simulink model "sim_tcst_2024_att_ctrl"  (R2020a)
settings: Solver=ode4  StartTime=0.0  StopTime=30.0  FixedStep=0.01  RelTol=1e-3
values from neighbouring files (symbols this model uses):
  beta0 = 2    [init_tcst_2024_att_ctrl.m]
  c1_diff_sigma_bar_w = diag([12; 12; 12])    [init_tcst_2024_att_ctrl.m]
  c1_diff_ui = diag([25; 30; 20])    [init_tcst_2024_att_ctrl.m]
  c2_diff_sigma_bar_w = diag([12; 12; 12])    [init_tcst_2024_att_ctrl.m]
  c2_diff_ui = diag([50; 50; 10])    [init_tcst_2024_att_ctrl.m]
  c3_diff_sigma_bar_w = diag([15; 15; 15])    [init_tcst_2024_att_ctrl.m]
  c3_diff_ui = diag([15; 15; 10])    [init_tcst_2024_att_ctrl.m]
  dw_aa_t = 0.2 * ones(3, 5) + ( 1.0 - 0.2 ) * rand(3, 5)    [init_tcst_2024_att_ctrl.m]
  dw_ff_t = [ 0.4 * ones(1, 5) + ( 1.0 - 0.4 ) * rand(1, 5);                      0.4 * ones(1, 5) + ( 1.0 - 0.4 ) * rand(1, 5);                      0.2 * ones(1, 5) + ( 0.6 - 0.2 ) * rand(1, 5) ]    [init_tcst_2024_att_ctrl.m]
  dw_phi_t = ( - pi / 2 ) * ones(3, 5) + ( pi / 2 - ( - pi / 2 ) ) * rand(3, 5)    [init_tcst_2024_att_ctrl.m]
  dwci_init = zeros(3,5)    [init_tcst_2024_att_ctrl.m]
  err_Ri_bar_init = zeros(3,NF)    [init_tcst_2024_att_ctrl.m]
  Fi_init = zeros(3,NF)    [init_tcst_2024_att_ctrl.m]
  h1w = diag([20.0; 20.0; 20.0])    [init_tcst_2024_att_ctrl.m]
  h2w = diag([30.0; 35.0; 35.0])    [init_tcst_2024_att_ctrl.m]
  h3w = diag([30.0; 25.0; 30.0])    [init_tcst_2024_att_ctrl.m]
  Ji = zeros(3,3,NF)    [init_tcst_2024_att_ctrl.m]
  kr1 = 10    [init_tcst_2024_att_ctrl.m]
  kr2 = 10    [init_tcst_2024_att_ctrl.m]
  kr3 = 5    [init_tcst_2024_att_ctrl.m]
  Lamd_diff_sigma_bar_w = 0.8    [init_tcst_2024_att_ctrl.m]
  Lamd_diff_ui = 0.8    [init_tcst_2024_att_ctrl.m]
  mu_d_w = 100    [init_tcst_2024_att_ctrl.m]
  pos0 = zeros(3, 1)    [init_tcst_2024_att_ctrl.m]
  PZ0 = P0(3)    [init_tcst_2024_att_ctrl.m]
  PZ1 = 10    [init_tcst_2024_att_ctrl.m]
  Qci_init = repmat([1;0;0;0],1,NF)    [init_tcst_2024_att_ctrl.m]
  Qei_init = zeros(4,NF)    [init_tcst_2024_att_ctrl.m]
  R0 = 4    [init_tcst_2024_att_ctrl.m]
  R1 = 8    [init_tcst_2024_att_ctrl.m]
  Rci_init = zeros(3,3,NF)    [init_tcst_2024_att_ctrl.m]
  Rei_init = zeros(3,3,NF)    [init_tcst_2024_att_ctrl.m]
  Ri_init = zeros(3,3,NF)    [init_tcst_2024_att_ctrl.m]
  Rx2 = 10    [init_tcst_2024_att_ctrl.m]
  Ry2 = 6    [init_tcst_2024_att_ctrl.m]
  Rz2 = 4    [init_tcst_2024_att_ctrl.m]
  T0 = 0    [init_tcst_2024_att_ctrl.m]
  T1 = tseq1    (= 10)    [init_tcst_2024_att_ctrl.m]
  T2 = tseq1 + tseq12 + tseq2    (= 30)    [init_tcst_2024_att_ctrl.m]
  ui_init = zeros(3,NF)    [init_tcst_2024_att_ctrl.m]
  V_Phi_Rei_init = zeros(3,NF)    [init_tcst_2024_att_ctrl.m]
  vel0 = zeros(3, 1)    [init_tcst_2024_att_ctrl.m]
  wci_init = zeros(3,5)    [init_tcst_2024_att_ctrl.m]
  wei_init = zeros(3,NF)    [init_tcst_2024_att_ctrl.m]
  zeta_diff_sigma_bar_w = 0.3    [init_tcst_2024_att_ctrl.m]
  zeta_diff_ui = 0.05    [init_tcst_2024_att_ctrl.m]
undefined symbols (not defined in the file or in its folder): cal_frac_squ, p_alfaw1, p_alfaw2, q_alfaw1, q_alfaw2, Qi_init, wi_init
(part 4 of 4)

== matlab function sim_tcst_2024_att_ctrl/cal dw_hat agent 3 ==
  data: h3w input; Ji input; d_sigma_bar_w_vec input; sigma_bar_w_hat_vec input; dw_hat_3 output
function dw_hat_3 = fcn(h3w, Ji, d_sigma_bar_w_vec, sigma_bar_w_hat_vec)
%%%% 计算扰动观测值dw_hat
iiuav = 3;
dw_hat_3 = Ji(:,:,iiuav) * d_sigma_bar_w_vec(:,iiuav) + h3w * sigma_bar_w_hat_vec(:,iiuav);

== matlab function sim_tcst_2024_att_ctrl/cal dw_hat agent 4 ==
  data: h3w input; Ji input; d_sigma_bar_w_vec input; sigma_bar_w_hat_vec input; dw_hat_4 output
function dw_hat_4 = fcn(h3w, Ji, d_sigma_bar_w_vec, sigma_bar_w_hat_vec)
%%%% 计算扰动观测值dw_hat
iiuav = 4;
dw_hat_4 = Ji(:,:,iiuav) * d_sigma_bar_w_vec(:,iiuav) + h3w * sigma_bar_w_hat_vec(:,iiuav);

== matlab function sim_tcst_2024_att_ctrl/cal dw_hat agent 5 ==
  data: h3w input; Ji input; d_sigma_bar_w_vec input; sigma_bar_w_hat_vec input; dw_hat_5 output
function dw_hat_5 = fcn(h3w, Ji, d_sigma_bar_w_vec, sigma_bar_w_hat_vec)
%%%% 计算扰动观测值dw_hat
iiuav = 5;
dw_hat_5 = Ji(:,:,iiuav) * d_sigma_bar_w_vec(:,iiuav) + h3w * sigma_bar_w_hat_vec(:,iiuav);

== matlab function sim_tcst_2024_att_ctrl/cal Fi agent 1 ==
  data: wei_vec input; Rei_vec input; Fi_1 output; wci_vec input; dwci_vec input
function Fi_1 = fcn(wei_vec, Rei_vec, wci_vec, dwci_vec)
%%%% 计算辅助姿态旋转误差
iiuav = 1;
Fi_1 = cal_askew_mat( wei_vec(:,iiuav) ) * ( Rei_vec(:,:,iiuav)' ) * wci_vec(:,iiuav) ...
            - ( Rei_vec(:,:,iiuav)' ) * dwci_vec(:,iiuav);
end

== matlab function sim_tcst_2024_att_ctrl/cal error dw_tilt ==
  data: dw_vec input; dw_hat_vec input; dw_tilt_vec output
function dw_tilt_vec = fcn(dw_vec, dw_hat_vec)
%%%% 计算扰动观测误差dw_tilt
dw_tilt_vec = zeros(3,5);
for iiuav = 1:5
    dw_tilt_vec(:,iiuav) = dw_vec(:,iiuav) - dw_hat_vec(:,iiuav);
end

== matlab function sim_tcst_2024_att_ctrl/cal sigma_bar_w_hat agent 1 ==
  data: h1w input; h2w input; theta_sigma_bar_w_tilt_1_vec input; d_sigma_bar_w_hat_1 output; theta_sigma_bar_w_tilt_2_vec input; d_sigma_bar_w_vec input
function d_sigma_bar_w_hat_1 = fcn(h1w, h2w, theta_sigma_bar_w_tilt_1_vec, theta_sigma_bar_w_tilt_2_vec, d_sigma_bar_w_vec)
%%%% 计算扰动观测器中虚拟速度控制量观测值sigma_w_hat的微分方程
iiuav = 1;
d_sigma_bar_w_hat_1 = d_sigma_bar_w_vec(:,iiuav) + ...
                                            h1w * theta_sigma_bar_w_tilt_1_vec(:,iiuav) + ...
                                            h2w * theta_sigma_bar_w_tilt_2_vec(:,iiuav);

== matlab function sim_tcst_2024_att_ctrl/cal sigma_bar_w_hat agent 2 ==
  data: h1w input; h2w input; theta_sigma_bar_w_tilt_1_vec input; d_sigma_bar_w_hat_2 output; theta_sigma_bar_w_tilt_2_vec input; d_sigma_bar_w_vec input
function d_sigma_bar_w_hat_2 = fcn(h1w, h2w, theta_sigma_bar_w_tilt_1_vec, theta_sigma_bar_w_tilt_2_vec, d_sigma_bar_w_vec)
%%%% 计算扰动观测器中虚拟速度控制量观测值sigma_v_hat的微分方程
iiuav = 2;
d_sigma_bar_w_hat_2 = d_sigma_bar_w_vec(:,iiuav) + ...
                                            h1w * theta_sigma_bar_w_tilt_1_vec(:,iiuav) + ...
                                            h2w * theta_sigma_bar_w_tilt_2_vec(:,iiuav);

== matlab function sim_tcst_2024_att_ctrl/cal sigma_bar_w_hat agent 3 ==
  data: h1w input; h2w input; theta_sigma_bar_w_tilt_1_vec input; d_sigma_bar_w_hat_3 output; theta_sigma_bar_w_tilt_2_vec input; d_sigma_bar_w_vec input
function d_sigma_bar_w_hat_3 = fcn(h1w, h2w, theta_sigma_bar_w_tilt_1_vec, theta_sigma_bar_w_tilt_2_vec, d_sigma_bar_w_vec)
%%%% 计算扰动观测器中虚拟速度控制量观测值sigma_w_hat的微分方程
iiuav = 3;
d_sigma_bar_w_hat_3 = d_sigma_bar_w_vec(:,iiuav) + ...
                                            h1w * theta_sigma_bar_w_tilt_1_vec(:,iiuav) + ...
                                            h2w * theta_sigma_bar_w_tilt_2_vec(:,iiuav);

== matlab function sim_tcst_2024_att_ctrl/cal sigma_bar_w_hat agent 4 ==
  data: h1w input; h2w input; theta_sigma_bar_w_tilt_1_vec input; d_sigma_bar_w_hat_4 output; theta_sigma_bar_w_tilt_2_vec input; d_sigma_bar_w_vec input
function d_sigma_bar_w_hat_4 = fcn(h1w, h2w, theta_sigma_bar_w_tilt_1_vec, theta_sigma_bar_w_tilt_2_vec, d_sigma_bar_w_vec)
%%%% 计算扰动观测器中虚拟速度控制量观测值sigma_w_hat的微分方程
iiuav = 4;
d_sigma_bar_w_hat_4 = d_sigma_bar_w_vec(:,iiuav) + ...
                                            h1w * theta_sigma_bar_w_tilt_1_vec(:,iiuav) + ...
                                            h2w * theta_sigma_bar_w_tilt_2_vec(:,iiuav);

== matlab function sim_tcst_2024_att_ctrl/cal sigma_bar_w_hat agent 5 ==
  data: h1w input; h2w input; theta_sigma_bar_w_tilt_1_vec input; d_sigma_bar_w_hat_5 output; theta_sigma_bar_w_tilt_2_vec input; d_sigma_bar_w_vec input
function d_sigma_bar_w_hat_5 = fcn(h1w, h2w, theta_sigma_bar_w_tilt_1_vec, theta_sigma_bar_w_tilt_2_vec, d_sigma_bar_w_vec)
%%%% 计算扰动观测器中虚拟速度控制量观测值sigma_w_hat的微分方程
iiuav = 5;
d_sigma_bar_w_hat_5 = d_sigma_bar_w_vec(:,iiuav) + ...
                                            h1w * theta_sigma_bar_w_tilt_1_vec(:,iiuav) + ...
                                            h2w * theta_sigma_bar_w_tilt_2_vec(:,iiuav);

== matlab function sim_tcst_2024_att_ctrl/cal sigma_w_bar ==
  data: sigma_bar_w_vec output; wi_vec input; sigma_w_vec input
function sigma_bar_w_vec = fcn(wi_vec, sigma_w_vec)
%%%% 计算姿态角速率跟踪误差
sigma_bar_w_vec = zeros(3,5);
for iiuav = 1:5
    sigma_bar_w_vec(:,iiuav) = wi_vec(:,iiuav) - sigma_w_vec(:,iiuav);
end

== matlab function sim_tcst_2024_att_ctrl/cal theta_sigma_bar_w_tilt agent 1 ==
  data: alfa_theta_obs_w input; sigma_bar_w_tilt_squ_1_1 input; theta_sigma_bar_w_tilt_1_1 output; sigma_bar_w_tilt_squ_2_1 input; sigma_bar_w_tilt_vec input; theta_sigma_bar_w_tilt_2_1 output
function [theta_sigma_bar_w_tilt_1_1, theta_sigma_bar_w_tilt_2_1] = fcn(alfa_theta_obs_w, sigma_bar_w_tilt_squ_1_1, sigma_bar_w_tilt_squ_2_1, sigma_bar_w_tilt_vec)
%%%% 计算平滑递增函数
iiuav = 1;
theta_sigma_bar_w_tilt_1_1 = sigma_bar_w_tilt_squ_1_1(:) .* ( -1 + 2 ./ ( 1 + exp( -alfa_theta_obs_w .* sigma_bar_w_tilt_vec(:,iiuav) ) ) );
theta_sigma_bar_w_tilt_2_1 = sigma_bar_w_tilt_squ_2_1(:) .* ( -1 + 2 ./ ( 1 + exp( -alfa_theta_obs_w .* sigma_bar_w_tilt_vec(:,iiuav) ) ) );

== matlab function sim_tcst_2024_att_ctrl/cal theta_sigma_bar_w_tilt agent 2 ==
  data: alfa_theta_obs_w input; sigma_bar_w_tilt_squ_1_2 input; theta_sigma_bar_w_tilt_1_2 output; sigma_bar_w_tilt_squ_2_2 input; sigma_bar_w_tilt_vec input; theta_sigma_bar_w_tilt_2_2 output
function [theta_sigma_bar_w_tilt_1_2, theta_sigma_bar_w_tilt_2_2] = fcn(alfa_theta_obs_w, sigma_bar_w_tilt_squ_1_2, sigma_bar_w_tilt_squ_2_2, sigma_bar_w_tilt_vec)
%%%% 计算平滑递增函数
iiuav = 2;
theta_sigma_bar_w_tilt_1_2 = sigma_bar_w_tilt_squ_1_2(:) .* ( -1 + 2 ./ ( 1 + exp( -alfa_theta_obs_w .* sigma_bar_w_tilt_vec(:,iiuav) ) ) );
theta_sigma_bar_w_tilt_2_2 = sigma_bar_w_tilt_squ_2_2(:) .* ( -1 + 2 ./ ( 1 + exp( -alfa_theta_obs_w .* sigma_bar_w_tilt_vec(:,iiuav) ) ) );

== matlab function sim_tcst_2024_att_ctrl/cal Fi agent 2 ==
  data: wei_vec input; Rei_vec input; Fi_2 output; wci_vec input; dwci_vec input
function Fi_2 = fcn(wei_vec, Rei_vec, wci_vec, dwci_vec)
%%%% 计算辅助姿态旋转误差
iiuav = 2;
Fi_2 = cal_askew_mat( wei_vec(:,iiuav) ) * ( Rei_vec(:,:,iiuav)' ) * wci_vec(:,iiuav) ...
            - ( Rei_vec(:,:,iiuav)' ) * dwci_vec(:,iiuav);
end

== matlab function sim_tcst_2024_att_ctrl/cal theta_sigma_bar_w_tilt agent 3 ==
  data: alfa_theta_obs_w input; sigma_bar_w_tilt_squ_1_3 input; theta_sigma_bar_w_tilt_1_3 output; sigma_bar_w_tilt_squ_2_3 input; sigma_bar_w_tilt_vec input; theta_sigma_bar_w_tilt_2_3 output
function [theta_sigma_bar_w_tilt_1_3, theta_sigma_bar_w_tilt_2_3] = fcn(alfa_theta_obs_w, sigma_bar_w_tilt_squ_1_3, sigma_bar_w_tilt_squ_2_3, sigma_bar_w_tilt_vec)
%%%% 计算平滑递增函数
iiuav = 3;
theta_sigma_bar_w_tilt_1_3 = sigma_bar_w_tilt_squ_1_3(:) .* ( -1 + 2 ./ ( 1 + exp( -alfa_theta_obs_w .* sigma_bar_w_tilt_vec(:,iiuav) ) ) );
theta_sigma_bar_w_tilt_2_3 = sigma_bar_w_tilt_squ_2_3(:) .* ( -1 + 2 ./ ( 1 + exp( -alfa_theta_obs_w .* sigma_bar_w_tilt_vec(:,iiuav) ) ) );

== matlab function sim_tcst_2024_att_ctrl/cal theta_sigma_bar_w_tilt agent 4 ==
  data: alfa_theta_obs_w input; sigma_bar_w_tilt_squ_1_4 input; theta_sigma_bar_w_tilt_1_4 output; sigma_bar_w_tilt_squ_2_4 input; sigma_bar_w_tilt_vec input; theta_sigma_bar_w_tilt_2_4 output
function [theta_sigma_bar_w_tilt_1_4, theta_sigma_bar_w_tilt_2_4] = fcn(alfa_theta_obs_w, sigma_bar_w_tilt_squ_1_4, sigma_bar_w_tilt_squ_2_4, sigma_bar_w_tilt_vec)
%%%% 计算平滑递增函数
iiuav = 4;
theta_sigma_bar_w_tilt_1_4 = sigma_bar_w_tilt_squ_1_4(:) .* ( -1 + 2 ./ ( 1 + exp( -alfa_theta_obs_w .* sigma_bar_w_tilt_vec(:,iiuav) ) ) );
theta_sigma_bar_w_tilt_2_4 = sigma_bar_w_tilt_squ_2_4(:) .* ( -1 + 2 ./ ( 1 + exp( -alfa_theta_obs_w .* sigma_bar_w_tilt_vec(:,iiuav) ) ) );

== matlab function sim_tcst_2024_att_ctrl/cal theta_sigma_bar_w_tilt agent 5 ==
  data: alfa_theta_obs_w input; sigma_bar_w_tilt_squ_1_5 input; theta_sigma_bar_w_tilt_1_5 output; sigma_bar_w_tilt_squ_2_5 input; sigma_bar_w_tilt_vec input; theta_sigma_bar_w_tilt_2_5 output
function [theta_sigma_bar_w_tilt_1_5, theta_sigma_bar_w_tilt_2_5] = fcn(alfa_theta_obs_w, sigma_bar_w_tilt_squ_1_5, sigma_bar_w_tilt_squ_2_5, sigma_bar_w_tilt_vec)
%%%% 计算平滑递增函数
iiuav = 5;
theta_sigma_bar_w_tilt_1_5 = sigma_bar_w_tilt_squ_1_5(:) .* ( -1 + 2 ./ ( 1 + exp( -alfa_theta_obs_w .* sigma_bar_w_tilt_vec(:,iiuav) ) ) );
theta_sigma_bar_w_tilt_2_5 = sigma_bar_w_tilt_squ_2_5(:) .* ( -1 + 2 ./ ( 1 + exp( -alfa_theta_obs_w .* sigma_bar_w_tilt_vec(:,iiuav) ) ) );

== matlab function sim_tcst_2024_att_ctrl/choose ksi_est_err 11 ==
  data: x input; y output
function y = fcn(x)
iiuav = 1;
y = x(:,iiuav);

== matlab function sim_tcst_2024_att_ctrl/choose ksi_est_err 12 ==
  data: x input; y output
function y = fcn(x)
iiuav = 1;
y = x(:,iiuav);

== matlab function sim_tcst_2024_att_ctrl/choose ksi_est_err 13 ==
  data: x input; y output
function y = fcn(x)
iiuav = 2;
y = x(:,iiuav);

== matlab function sim_tcst_2024_att_ctrl/choose ksi_est_err 14 ==
  data: x input; y output
function y = fcn(x)
iiuav = 2;
y = x(:,iiuav);

== matlab function sim_tcst_2024_att_ctrl/choose ksi_est_err 15 ==
  data: x input; y output
function y = fcn(x)
iiuav = 3;
y = x(:,iiuav);

== matlab function sim_tcst_2024_att_ctrl/choose ksi_est_err 16 ==
  data: x input; y output
function y = fcn(x)
iiuav = 3;
y = x(:,iiuav);

== matlab function sim_tcst_2024_att_ctrl/choose ksi_est_err 17 ==
  data: x input; y output
function y = fcn(x)
iiuav = 4;
y = x(:,iiuav);

== matlab function sim_tcst_2024_att_ctrl/choose ksi_est_err 18 ==
  data: x input; y output
function y = fcn(x)
iiuav = 4;
y = x(:,iiuav);

== matlab function sim_tcst_2024_att_ctrl/choose ksi_est_err 19 ==
  data: x input; y output
function y = fcn(x)
iiuav = 5;
y = x(:,iiuav);

== matlab function sim_tcst_2024_att_ctrl/choose ksi_est_err 20 ==
  data: x input; y output
function y = fcn(x)
iiuav = 5;
y = x(:,iiuav);

== matlab function sim_tcst_2024_att_ctrl/cal Fi agent 3 ==
  data: wei_vec input; Rei_vec input; Fi_3 output; wci_vec input; dwci_vec input
function Fi_3 = fcn(wei_vec, Rei_vec, wci_vec, dwci_vec)
%%%% 计算辅助姿态旋转误差
iiuav = 3;
Fi_3 = cal_askew_mat( wei_vec(:,iiuav) ) * ( Rei_vec(:,:,iiuav)' ) * wci_vec(:,iiuav) ...
            - ( Rei_vec(:,:,iiuav)' ) * dwci_vec(:,iiuav);
end

== matlab function sim_tcst_2024_att_ctrl/combine d_sigma_bar_v_est ==
  data: d_sigma_bar_w_est_1 input; d_sigma_bar_w_est_2 input; d_sigma_bar_w_est_3 input; d_sigma_bar_w_est_4 input; d_sigma_bar_w_est_5 input; d_sigma_bar_w_vec output
function d_sigma_bar_w_vec  = fcn(d_sigma_bar_w_est_1, d_sigma_bar_w_est_2, d_sigma_bar_w_est_3, d_sigma_bar_w_est_4, d_sigma_bar_w_est_5)
%%%% 合并用微分器求得的虚拟速度控制量导数
d_sigma_bar_w_vec = [d_sigma_bar_w_est_1(:), d_sigma_bar_w_est_2(:), d_sigma_bar_w_est_3(:), d_sigma_bar_w_est_4(:), d_sigma_bar_w_est_5(:)];

== matlab function sim_tcst_2024_att_ctrl/combine dw_hat ==
  data: dw_hat_1 input; dw_hat_2 input; dw_hat_3 input; dw_hat_4 input; dw_hat_5 input; dw_hat_vec output
function dw_hat_vec  = fcn(dw_hat_1, dw_hat_2, dw_hat_3, dw_hat_4, dw_hat_5)
%%%% 合并扰动观测值dw_hat
dw_hat_vec = [dw_hat_1(:), dw_hat_2(:), dw_hat_3(:), dw_hat_4(:), dw_hat_5(:)];

== matlab function sim_tcst_2024_att_ctrl/combine sigma_bar_w_hat ==
  data: sigma_bar_w_hat_1 input; sigma_bar_w_hat_2 input; sigma_bar_w_hat_3 input; sigma_bar_w_hat_4 input; sigma_bar_w_hat_5 input; sigma_bar_w_hat_vec output
function sigma_bar_w_hat_vec  = fcn(sigma_bar_w_hat_1, sigma_bar_w_hat_2, sigma_bar_w_hat_3, sigma_bar_w_hat_4, sigma_bar_w_hat_5)
%%%% 合并虚拟速度控制量观测值sigma_bar_w_hat
sigma_bar_w_hat_vec = [sigma_bar_w_hat_1(:), sigma_bar_w_hat_2(:), sigma_bar_w_hat_3(:), sigma_bar_w_hat_4(:), sigma_bar_w_hat_5(:)];

== matlab function sim_tcst_2024_att_ctrl/combine sigma_w ==
  data: sigma_w_1 input; sigma_w_vec output; sigma_w_2 input; sigma_w_3 input; sigma_w_4 input; sigma_w_5 input
function sigma_w_vec = fcn(sigma_w_1, sigma_w_2, sigma_w_3, sigma_w_4, sigma_w_5)
%%%% 合并辅助姿态角速率
sigma_w_vec = [sigma_w_1(:), sigma_w_2(:), sigma_w_3(:), sigma_w_4(:), sigma_w_5(:)];

== matlab function sim_tcst_2024_att_ctrl/combine theta_sigma_bar_w_tilt ==
  data: theta_sigma_bar_w_tilt_1_1 input; theta_sigma_bar_w_tilt_1_2 input; theta_sigma_bar_w_tilt_1_3 input; theta_sigma_bar_w_tilt_1_4 input; theta_sigma_bar_w_tilt_1_5 input; theta_sigma_bar_w_tilt_1_vec output; theta_sigma_bar_w_tilt_2_1 input; theta_sigma_bar_w_tilt_2_vec output; theta_sigma_bar_w_tilt_2_2 input; theta_sigma_bar_w_tilt_2_3 input; theta_sigma_bar_w_tilt_2_4 input; theta_sigma_bar_w_tilt_2_5 input
function [theta_sigma_bar_w_tilt_1_vec, theta_sigma_bar_w_tilt_2_vec]  = fcn(theta_sigma_bar_w_tilt_1_1, theta_sigma_bar_w_tilt_1_2, theta_sigma_bar_w_tilt_1_3, theta_sigma_bar_w_tilt_1_4, theta_sigma_bar_w_tilt_1_5, ...
                                                                                                                                            theta_sigma_bar_w_tilt_2_1, theta_sigma_bar_w_tilt_2_2, theta_sigma_bar_w_tilt_2_3, theta_sigma_bar_w_tilt_2_4, theta_sigma_bar_w_tilt_2_5)
%%%% 合并领导者位置观测器输出结果
theta_sigma_bar_w_tilt_1_vec = [theta_sigma_bar_w_tilt_1_1(:), theta_sigma_bar_w_tilt_1_2(:), theta_sigma_bar_w_tilt_1_3(:), theta_sigma_bar_w_tilt_1_4(:), theta_sigma_bar_w_tilt_1_5(:)];
theta_sigma_bar_w_tilt_2_vec = [theta_sigma_bar_w_tilt_2_1(:), theta_sigma_bar_w_tilt_2_2(:), theta_sigma_bar_w_tilt_2_3(:), theta_sigma_bar_w_tilt_2_4(:), theta_sigma_bar_w_tilt_2_5(:)];

== matlab function sim_tcst_2024_att_ctrl/trans to column51 ==
  data: x input; y output
function y = fcn(x)
y = x(:);

== matlab function sim_tcst_2024_att_ctrl/trans to column52 ==
  data: x input; y output
function y = fcn(x)
y = x(:);

== matlab function sim_tcst_2024_att_ctrl/trans to column53 ==
  data: x input; y output
function y = fcn(x)
y = x(:);

== matlab function sim_tcst_2024_att_ctrl/trans to column54 ==
  data: x input; y output
function y = fcn(x)
y = x(:);

== matlab function sim_tcst_2024_att_ctrl/trans to column55 ==
  data: x input; y output
function y = fcn(x)
y = x(:);

== matlab function sim_tcst_2024_att_ctrl/trans to column56 ==
  data: x input; y output
function y = fcn(x)
y = x(:);

== matlab function sim_tcst_2024_att_ctrl/cal Fi agent 4 ==
  data: wei_vec input; Rei_vec input; Fi_4 output; wci_vec input; dwci_vec input
function Fi_4 = fcn(wei_vec, Rei_vec, wci_vec, dwci_vec)
%%%% 计算辅助姿态旋转误差
iiuav = 4;
Fi_4 = cal_askew_mat( wei_vec(:,iiuav) ) * ( Rei_vec(:,:,iiuav)' ) * wci_vec(:,iiuav) ...
            - ( Rei_vec(:,:,iiuav)' ) * dwci_vec(:,iiuav);
end

== matlab function sim_tcst_2024_att_ctrl/trans to column57 ==
  data: x input; y output
function y = fcn(x)
y = x(:);

== matlab function sim_tcst_2024_att_ctrl/trans to column58 ==
  data: x input; y output
function y = fcn(x)
y = x(:);

== matlab function sim_tcst_2024_att_ctrl/trans to column59 ==
  data: x input; y output
function y = fcn(x)
y = x(:);

== matlab function sim_tcst_2024_att_ctrl/trans to column60 ==
  data: x input; y output
function y = fcn(x)
y = x(:);

== matlab function sim_tcst_2024_att_ctrl/combine tau1 ==
  data: dw_1 input; dw_vec output; dw_2 input; dw_3 input; dw_4 input; dw_5 input
function dw_vec = fcn(dw_1, dw_2, dw_3, dw_4, dw_5)
%%%% 合并辅助姿态角速率
dw_vec = [dw_1(:), dw_2(:), dw_3(:), dw_4(:), dw_5(:)];

== matlab function sim_tcst_2024_att_ctrl/generate angular rate disturbance agent 1 ==
  data: dw_1 output; dw_aa_t input; dw_ff_t input; dw_phi_t input; t input
function dw_1 = fcn(dw_aa_t, dw_ff_t, dw_phi_t, t)
%%%% 姿态动力学方程中的扰动项设置
epsil_t = zeros(3, 1);

for kk = 1:5
    epsil_t = epsil_t + dw_aa_t(:, kk) .* sin( 2 * pi * dw_ff_t(:, kk) * t + dw_phi_t(:, kk) );
end

dw_1 = [ epsil_t(1) + 1.6 * sin( 0.4 * t ) + 2.0 * cos( 0.5 * t ) + 1.4 * sin( 0.7 * t ) ...
                + 4 * exp( -0.1 * t ) * sin( 0.8 * t ) + 3 / ( 1 + exp( -0.2 * ( t - 15 ) ) ); ...
                epsil_t(2) + 1.2 * sin( 0.2 * t ) + 3 * cos( 0.4 * t ) + 0.8 * sin( 0.6 * t ) ...
                + 2 * exp( -0.15 * t ) * cos( 1.2 * t ) + 3 / ( 1 + exp( -0.3 * ( t - 25 ) ) ); ...
                epsil_t(3) + 1.8 * sin( 0.2 * t ) + 1.6 * sin( 0.3 * t ) + 1.6 * cos( 0.4 * t ) ...
                + 4 * exp( -0.05 * t ) * sin( 0.5 * t + pi / 4 ) + 3 / ( 1 + exp( -0.5 * ( t - 20 ) ) ) ];

== matlab function sim_tcst_2024_att_ctrl/generate angular rate disturbance agent 2 ==
  data: dw_2 output; dw_aa_t input; dw_ff_t input; dw_phi_t input; t input
function dw_2 = fcn(dw_aa_t, dw_ff_t, dw_phi_t, t)
%%%% 姿态动力学方程中的扰动项设置
epsil_t = zeros(3, 1);

for kk = 1:5
    epsil_t = epsil_t + dw_aa_t(:, kk) .* sin( 2 * pi * dw_ff_t(:, kk) * t + dw_phi_t(:, kk) );
end

dw_2 = [ epsil_t(1) + 1.6 * sin( 0.2 * t ) + 2.0 * cos( 0.3 * t ) + 1.4 * sin( 0.5 * t ) ...
                + 4 * exp( -0.1 * t ) * sin( 0.5 * t ) + 3 / ( 1 + exp( -0.2 * ( t - 15 ) ) ); ...
                epsil_t(2) + 1.2 * sin( 0.1 * t ) + 3 * cos( 0.2 * t ) + 0.8 * sin( 0.4 * t ) ...
                + 2 * exp( -0.15 * t ) * cos( 0.6 * t ) + 3 / ( 1 + exp( -0.3 * ( t - 25 ) ) ); ...
                epsil_t(3) + 1.8 * sin( 0.1 * t ) + 1.6 * sin( 0.2 * t ) + 1.6 * cos( 0.3 * t ) ...
                + 4 * exp( -0.05 * t ) * sin( 0.4 * t + pi / 4 ) + 3 / ( 1 + exp( -0.5 * ( t - 20 ) ) ) ];

== matlab function sim_tcst_2024_att_ctrl/generate angular rate disturbance agent 3 ==
  data: dw_3 output; dw_aa_t input; dw_ff_t input; dw_phi_t input; t input
function dw_3 = fcn(dw_aa_t, dw_ff_t, dw_phi_t, t)
%%%% 姿态动力学方程中的扰动项设置
epsil_t = zeros(3, 1);

for kk = 1:5
    epsil_t = epsil_t + dw_aa_t(:, kk) .* sin( 2 * pi * dw_ff_t(:, kk) * t + dw_phi_t(:, kk) );
end

dw_3 = [ epsil_t(1) + 1.6 * sin( 0.2 * t ) + 2.0 * cos( 0.3 * t ) + 1.4 * sin( 0.5 * t ) ...
                + 4 * exp( -0.1 * t ) * sin( 0.5 * t ) + 3 / ( 1 + exp( -0.2 * ( t - 15 ) ) ); ...
                epsil_t(2) + 1.2 * sin( 0.1 * t ) + 3 * cos( 0.2 * t ) + 0.8 * sin( 0.4 * t ) ...
                + 2 * exp( -0.15 * t ) * cos( 0.6 * t ) + 3 / ( 1 + exp( -0.3 * ( t - 25 ) ) ); ...
                epsil_t(3) + 1.8 * sin( 0.1 * t ) + 1.6 * sin( 0.2 * t ) + 1.6 * cos( 0.3 * t ) ...
                + 4 * exp( -0.05 * t ) * sin( 0.4 * t + pi / 4 ) + 3 / ( 1 + exp( -0.5 * ( t - 20 ) ) ) ];

== matlab function sim_tcst_2024_att_ctrl/generate angular rate disturbance agent 4 ==
  data: dw_4 output; dw_aa_t input; dw_ff_t input; dw_phi_t input; t input
function dw_4 = fcn(dw_aa_t, dw_ff_t, dw_phi_t, t)
%%%% 姿态动力学方程中的扰动项设置
epsil_t = zeros(3, 1);

for kk = 1:5
    epsil_t = epsil_t + dw_aa_t(:, kk) .* sin( 2 * pi * dw_ff_t(:, kk) * t + dw_phi_t(:, kk) );
end

dw_4 = [ epsil_t(1) + 1.6 * sin( 0.2 * t ) + 2.0 * cos( 0.3 * t ) + 1.4 * sin( 0.5 * t ) ...
                + 4 * exp( -0.1 * t ) * sin( 0.5 * t ) + 3 / ( 1 + exp( -0.2 * ( t - 15 ) ) ); ...
                epsil_t(2) + 1.2 * sin( 0.1 * t ) + 3 * cos( 0.2 * t ) + 0.8 * sin( 0.4 * t ) ...
                + 2 * exp( -0.15 * t ) * cos( 0.6 * t ) + 3 / ( 1 + exp( -0.3 * ( t - 25 ) ) ); ...
                epsil_t(3) + 1.8 * sin( 0.1 * t ) + 1.6 * sin( 0.2 * t ) + 1.6 * cos( 0.3 * t ) ...
                + 4 * exp( -0.05 * t ) * sin( 0.4 * t + pi / 4 ) + 3 / ( 1 + exp( -0.5 * ( t - 20 ) ) ) ];

== matlab function sim_tcst_2024_att_ctrl/generate angular rate disturbance agent 5 ==
  data: dw_5 output; dw_aa_t input; dw_ff_t input; dw_phi_t input; t input
function dw_5 = fcn(dw_aa_t, dw_ff_t, dw_phi_t, t)
%%%% 姿态动力学方程中的扰动项设置
epsil_t = zeros(3, 1);

for kk = 1:5
    epsil_t = epsil_t + dw_aa_t(:, kk) .* sin( 2 * pi * dw_ff_t(:, kk) * t + dw_phi_t(:, kk) );
end

dw_5 = [ epsil_t(1) + 1.6 * sin( 0.2 * t ) + 2.0 * cos( 0.3 * t ) + 1.4 * sin( 0.5 * t ) ...
                + 4 * exp( -0.1 * t ) * sin( 0.5 * t ) + 3 / ( 1 + exp( -0.2 * ( t - 15 ) ) ); ...
                epsil_t(2) + 1.2 * sin( 0.1 * t ) + 3 * cos( 0.2 * t ) + 0.8 * sin( 0.4 * t ) ...
                + 2 * exp( -0.15 * t ) * cos( 0.6 * t ) + 3 / ( 1 + exp( -0.3 * ( t - 25 ) ) ); ...
                epsil_t(3) + 1.8 * sin( 0.1 * t ) + 1.6 * sin( 0.2 * t ) + 1.6 * cos( 0.3 * t ) ...
                + 4 * exp( -0.05 * t ) * sin( 0.4 * t + pi / 4 ) + 3 / ( 1 + exp( -0.5 * ( t - 20 ) ) ) ];

== matlab function sim_tcst_2024_att_ctrl/combine norminal formation control input ==
  data: ui_1 input; ui_vec output; ui_2 input; ui_3 input; ui_4 input; ui_5 input
function ui_vec = fcn(ui_1, ui_2, ui_3, ui_4, ui_5)
%%%% 合并领导者编队跟踪误差结果
ui_vec = [ui_1(:), ui_2(:), ui_3(:), ui_4(:), ui_5(:)];

== matlab function sim_tcst_2024_att_ctrl/cal Fi agent 5 ==
  data: wei_vec input; Rei_vec input; Fi_5 output; wci_vec input; dwci_vec input
function Fi_5 = fcn(wei_vec, Rei_vec, wci_vec, dwci_vec)
%%%% 计算辅助姿态旋转误差
iiuav = 5;
Fi_5 = cal_askew_mat( wei_vec(:,iiuav) ) * ( Rei_vec(:,:,iiuav)' ) * wci_vec(:,iiuav) ...
            - ( Rei_vec(:,:,iiuav)' ) * dwci_vec(:,iiuav);
end

== matlab function sim_tcst_2024_att_ctrl/control input generator agent 1 ==
  data: u0 input; ui output
function ui  = fcn(u0)
%%%% 给出领导者参考加速度控制输入
g0 = 9.80663;
e3 = [0;0;1];

ui = g0 * e3 + u0(:);

== matlab function sim_tcst_2024_att_ctrl/control input generator agent 2 ==
  data: u0 input; ui output
function ui  = fcn(u0)
%%%% 给出领导者参考加速度控制输入
g0 = 9.80663;
e3 = [0;0;1];

ui = g0 * e3 + u0(:);

== matlab function sim_tcst_2024_att_ctrl/control input generator agent 3 ==
  data: u0 input; ui output
function ui  = fcn(u0)
%%%% 给出领导者参考加速度控制输入
g0 = 9.80663;
e3 = [0;0;1];

ui = g0 * e3 + u0(:);

== matlab function sim_tcst_2024_att_ctrl/control input generator agent 4 ==
  data: u0 input; ui output
function ui  = fcn(u0)
%%%% 给出领导者参考加速度控制输入
g0 = 9.80663;
e3 = [0;0;1];

ui = g0 * e3 + u0(:);

== matlab function sim_tcst_2024_att_ctrl/control input generator agent 5 ==
  data: u0 input; ui output
function ui  = fcn(u0)
%%%% 给出领导者参考加速度控制输入
g0 = 9.80663;
e3 = [0;0;1];

ui = g0 * e3 + u0(:);

== matlab function sim_tcst_2024_att_ctrl/combine err_Ri_bar1 ==
  data: Fi_1 input; Fi_vec output; Fi_2 input; Fi_3 input; Fi_4 input; Fi_5 input
function Fi_vec = fcn(Fi_1, Fi_2, Fi_3, Fi_4, Fi_5)
%%%% 合并补偿函数向量
Fi_vec = [Fi_1(:), Fi_2(:), Fi_3(:), Fi_4(:), Fi_5(:)];

== matlab function sim_tcst_2024_att_ctrl/update VTi agent 1 ==
  data: kr2 input; kr3 input; d_VTi_1 output; beta0 input; err_Ri_bar_vec input
function d_VTi_1 = fcn(kr2, kr3, beta0, err_Ri_bar_vec)
%%%% 更新非线性Filippov解向量
iiuav = 1;
d_VTi_1 = kr3 * kr2 * err_Ri_bar_vec(:,iiuav) - beta0 * sign( err_Ri_bar_vec(:,iiuav) );
end

== matlab function sim_tcst_2024_att_ctrl/update VTi agent 2 ==
  data: kr2 input; kr3 input; d_VTi_2 output; beta0 input; err_Ri_bar_vec input
function d_VTi_2 = fcn(kr2, kr3, beta0, err_Ri_bar_vec)
%%%% 更新非线性Filippov解向量
iiuav = 2;
d_VTi_2 = kr3 * kr2 * err_Ri_bar_vec(:,iiuav) - beta0 * sign( err_Ri_bar_vec(:,iiuav) );
end

== matlab function sim_tcst_2024_att_ctrl/update VTi agent 3 ==
  data: kr2 input; kr3 input; d_VTi_3 output; beta0 input; err_Ri_bar_vec input
function d_VTi_3 = fcn(kr2, kr3, beta0, err_Ri_bar_vec)
%%%% 更新非线性Filippov解向量
iiuav = 3;
d_VTi_3 = kr3 * kr2 * err_Ri_bar_vec(:,iiuav) - beta0 * sign( err_Ri_bar_vec(:,iiuav) );
end

== matlab function sim_tcst_2024_att_ctrl/update VTi agent 4 ==
  data: kr2 input; kr3 input; d_VTi_4 output; beta0 input; err_Ri_bar_vec input
function d_VTi_4 = fcn(kr2, kr3, beta0, err_Ri_bar_vec)
%%%% 更新非线性Filippov解向量
iiuav = 4;
d_VTi_4 = kr3 * kr2 * err_Ri_bar_vec(:,iiuav) - beta0 * sign( err_Ri_bar_vec(:,iiuav) );
end

== matlab function sim_tcst_2024_att_ctrl/update VTi agent 5 ==
  data: kr2 input; kr3 input; d_VTi_5 output; beta0 input; err_Ri_bar_vec input
function d_VTi_5 = fcn(kr2, kr3, beta0, err_Ri_bar_vec)
%%%% 更新非线性Filippov解向量
iiuav = 5;
d_VTi_5 = kr3 * kr2 * err_Ri_bar_vec(:,iiuav) - beta0 * sign( err_Ri_bar_vec(:,iiuav) );
end

== matlab function sim_tcst_2024_att_ctrl/combine VTi ==
  data: VTi_1 input; VTi_vec output; VTi_2 input; VTi_3 input; VTi_4 input; VTi_5 input
function VTi_vec = fcn(VTi_1, VTi_2, VTi_3, VTi_4, VTi_5)
%%%% 合并非线性Filippov解向量
VTi_vec = [VTi_1(:), VTi_2(:), VTi_3(:), VTi_4(:), VTi_5(:)];

== matlab function sim_tcst_2024_att_ctrl/cal taui agent 2 ==
  data: kr1 input; kr2 input; kr3 input; tau_2 output; Ji input; wi_vec input; wei_vec input; err_Ri_bar_vec input; Fi_vec input; VTi_vec input; dw_hat_vec input
function tau_2 = fcn(kr1, kr2, kr3, Ji, wi_vec, wei_vec, err_Ri_bar_vec, Fi_vec, VTi_vec, dw_hat_vec)
%%%% 计算用于姿态控制的驱动力矩控制输入
iiuav = 2;
tau_2 = -( kr3 + kr2 ) * err_Ri_bar_vec(:,iiuav) - kr1 * Ji(:,:,iiuav) * wei_vec(:,iiuav) ...
                + cal_askew_mat( wi_vec(:,iiuav) ) * Ji(:,:,iiuav) * wi_vec(:,iiuav) ...
                - Ji(:,:,iiuav) * Fi_vec(:,iiuav) - dw_hat_vec(:,iiuav) - VTi_vec(:,iiuav);
end

== matlab function sim_tcst_2024_att_ctrl/cal taui agent 3 ==
  data: kr1 input; kr2 input; kr3 input; tau_3 output; Ji input; wi_vec input; wei_vec input; err_Ri_bar_vec input; Fi_vec input; VTi_vec input; dw_hat_vec input
function tau_3 = fcn(kr1, kr2, kr3, Ji, wi_vec, wei_vec, err_Ri_bar_vec, Fi_vec, VTi_vec, dw_hat_vec)
%%%% 计算用于姿态控制的驱动力矩控制输入
iiuav = 3;
tau_3 = -( kr3 + kr2 ) * err_Ri_bar_vec(:,iiuav) - kr1 * Ji(:,:,iiuav) * wei_vec(:,iiuav) ...
                + cal_askew_mat( wi_vec(:,iiuav) ) * Ji(:,:,iiuav) * wi_vec(:,iiuav) ...
                - Ji(:,:,iiuav) * Fi_vec(:,iiuav) - dw_hat_vec(:,iiuav) - VTi_vec(:,iiuav);
end

== matlab function sim_tcst_2024_att_ctrl/cal taui agent 4 ==
  data: kr1 input; kr2 input; kr3 input; tau_4 output; Ji input; wi_vec input; wei_vec input; err_Ri_bar_vec input; Fi_vec input; VTi_vec input; dw_hat_vec input
function tau_4 = fcn(kr1, kr2, kr3, Ji, wi_vec, wei_vec, err_Ri_bar_vec, Fi_vec, VTi_vec, dw_hat_vec)
%%%% 计算用于姿态控制的驱动力矩控制输入
iiuav = 4;
tau_4 = -( kr3 + kr2 ) * err_Ri_bar_vec(:,iiuav) - kr1 * Ji(:,:,iiuav) * wei_vec(:,iiuav) ...
                + cal_askew_mat( wi_vec(:,iiuav) ) * Ji(:,:,iiuav) * wi_vec(:,iiuav) ...
                - Ji(:,:,iiuav) * Fi_vec(:,iiuav) - dw_hat_vec(:,iiuav) - VTi_vec(:,iiuav);
end

== matlab function sim_tcst_2024_att_ctrl/cal taui agent 5 ==
  data: kr1 input; kr2 input; kr3 input; tau_5 output; Ji input; wi_vec input; wei_vec input; err_Ri_bar_vec input; Fi_vec input; VTi_vec input; dw_hat_vec input
function tau_5 = fcn(kr1, kr2, kr3, Ji, wi_vec, wei_vec, err_Ri_bar_vec, Fi_vec, VTi_vec, dw_hat_vec)
%%%% 计算用于姿态控制的驱动力矩控制输入
iiuav = 5;
tau_5 = -( kr3 + kr2 ) * err_Ri_bar_vec(:,iiuav) - kr1 * Ji(:,:,iiuav) * wei_vec(:,iiuav) ...
                + cal_askew_mat( wi_vec(:,iiuav) ) * Ji(:,:,iiuav) * wi_vec(:,iiuav) ...
                - Ji(:,:,iiuav) * Fi_vec(:,iiuav) - dw_hat_vec(:,iiuav) - VTi_vec(:,iiuav);
end

== matlab function sim_tcst_2024_att_ctrl/depart err_Ri_bar 5 ==
  data: y output; x input
function y = fcn(x)
y = x(:,5);

end

== matlab function sim_tcst_2024_att_ctrl/cal d_theta_hat ==
  data: c1 input; d_ui_hat output; d_dui_hat output; d_d2ui_hat output; c2 input; c3 input; chi_t input; ui_sig_1 input; ui_sig_2 input; ui_sig_3 input; ui_sig_4 input; ui_sig_5 input; ui_sig_6 input; dui_hat input; d2ui_hat input
function [d_ui_hat, d_dui_hat, d_d2ui_hat] = fcn(c1, c2, c3, chi_t, ui_sig_1, ui_sig_2, ui_sig_3, ...
                                                                                        ui_sig_4, ui_sig_5, ui_sig_6, dui_hat, d2ui_hat)
d_d2ui_hat = -chi_t .* c1 * ui_sig_1(:) - (1 - chi_t) .* c1 * ui_sig_2(:);
d_dui_hat = -chi_t .* c2 * ui_sig_3(:) - (1 - chi_t) .* c2 * ui_sig_4(:) + d2ui_hat(:);
d_ui_hat = -chi_t .* c3 * ui_sig_5(:) - (1 - chi_t) .* c3 * ui_sig_6(:) + dui_hat(:);

== matlab function sim_tcst_2024_att_ctrl/depart err_Ri_bar 1 ==
  data: y output; x input
function y = fcn(x)
y = x(:,1);

end

== matlab function sim_tcst_2024_att_ctrl/cal sig ==
  data: x input; z output; y input
function z = fcn(x, y)
z = x(:) .* sign(y(:));

== matlab function sim_tcst_2024_att_ctrl/cal sig1 ==
  data: x input; z output; y input
function z = fcn(x, y)
z = x(:) .* sign(y(:));

== matlab function sim_tcst_2024_att_ctrl/cal sig2 ==
  data: x input; z output; y input
function z = fcn(x, y)
z = x(:) .* sign(y(:));

== matlab function sim_tcst_2024_att_ctrl/cal sig3 ==
  data: x input; z output; y input
function z = fcn(x, y)
z = x(:) .* sign(y(:));

== matlab function sim_tcst_2024_att_ctrl/cal sig4 ==
  data: x input; z output; y input
function z = fcn(x, y)
z = x(:) .* sign(y(:));

== matlab function sim_tcst_2024_att_ctrl/cal sig5 ==
  data: x input; z output; y input
function z = fcn(x, y)
z = x(:) .* sign(y(:));

== matlab function sim_tcst_2024_att_ctrl/trans to column10 ==
  data: x input; y output
function y = fcn(x)
y = x(:);

== matlab function sim_tcst_2024_att_ctrl/trans to column5 ==
  data: x input; y output
function y = fcn(x)
y = x(:);

== matlab function sim_tcst_2024_att_ctrl/trans to column6 ==
  data: x input; y output
function y = fcn(x)
y = x(:);

== matlab function sim_tcst_2024_att_ctrl/trans to column7 ==
  data: x input; y output
function y = fcn(x)
y = x(:);

== matlab function sim_tcst_2024_att_ctrl/trans to column8 ==
  data: x input; y output
function y = fcn(x)
y = x(:);

== matlab function sim_tcst_2024_att_ctrl/trans to column9 ==
  data: x input; y output
function y = fcn(x)
y = x(:);

== matlab function sim_tcst_2024_att_ctrl/choose ui agent 1 ==
  data: x input; y output
function y = fcn(x)
iiuav = 1;
y = x(:,iiuav);

== matlab function sim_tcst_2024_att_ctrl/cal d_theta_hat1 ==
  data: c1 input; d_ui_hat output; d_dui_hat output; d_d2ui_hat output; c2 input; c3 input; chi_t input; ui_sig_1 input; ui_sig_2 input; ui_sig_3 input; ui_sig_4 input; ui_sig_5 input; ui_sig_6 input; dui_hat input; d2ui_hat input
function [d_ui_hat, d_dui_hat, d_d2ui_hat] = fcn(c1, c2, c3, chi_t, ui_sig_1, ui_sig_2, ui_sig_3, ...
                                                                                        ui_sig_4, ui_sig_5, ui_sig_6, dui_hat, d2ui_hat)
d_d2ui_hat = -chi_t .* c1 * ui_sig_1(:) - (1 - chi_t) .* c1 * ui_sig_2(:);
d_dui_hat = -chi_t .* c2 * ui_sig_3(:) - (1 - chi_t) .* c2 * ui_sig_4(:) + d2ui_hat(:);
d_ui_hat = -chi_t .* c3 * ui_sig_5(:) - (1 - chi_t) .* c3 * ui_sig_6(:) + dui_hat(:);

== matlab function sim_tcst_2024_att_ctrl/cal sig10 ==
  data: x input; z output; y input
function z = fcn(x, y)
z = x(:) .* sign(y(:));

== matlab function sim_tcst_2024_att_ctrl/cal sig11 ==
  data: x input; z output; y input
function z = fcn(x, y)
z = x(:) .* sign(y(:));

== matlab function sim_tcst_2024_att_ctrl/cal sig6 ==
  data: x input; z output; y input
function z = fcn(x, y)
z = x(:) .* sign(y(:));

== matlab function sim_tcst_2024_att_ctrl/cal sig7 ==
  data: x input; z output; y input
function z = fcn(x, y)
z = x(:) .* sign(y(:));

== matlab function sim_tcst_2024_att_ctrl/cal sig8 ==
  data: x input; z output; y input
function z = fcn(x, y)
z = x(:) .* sign(y(:));

== matlab function sim_tcst_2024_att_ctrl/cal sig9 ==
  data: x input; z output; y input
function z = fcn(x, y)
z = x(:) .* sign(y(:));

== matlab function sim_tcst_2024_att_ctrl/choose ui agent 2 ==
  data: x input; y output
function y = fcn(x)
iiuav = 2;
y = x(:,iiuav);

== matlab function sim_tcst_2024_att_ctrl/trans to column11 ==
  data: x input; y output
function y = fcn(x)
y = x(:);

== matlab function sim_tcst_2024_att_ctrl/trans to column12 ==
  data: x input; y output
function y = fcn(x)
y = x(:);

== matlab function sim_tcst_2024_att_ctrl/trans to column13 ==
  data: x input; y output
function y = fcn(x)
y = x(:);

== matlab function sim_tcst_2024_att_ctrl/trans to column14 ==
  data: x input; y output
function y = fcn(x)
y = x(:);

== matlab function sim_tcst_2024_att_ctrl/trans to column15 ==
  data: x input; y output
function y = fcn(x)
y = x(:);

== matlab function sim_tcst_2024_att_ctrl/trans to column16 ==
  data: x input; y output
function y = fcn(x)
y = x(:);

== matlab function sim_tcst_2024_att_ctrl/cal d_theta_hat2 ==
  data: c1 input; d_ui_hat output; d_dui_hat output; d_d2ui_hat output; c2 input; c3 input; chi_t input; ui_sig_1 input; ui_sig_2 input; ui_sig_3 input; ui_sig_4 input; ui_sig_5 input; ui_sig_6 input; dui_hat input; d2ui_hat input
function [d_ui_hat, d_dui_hat, d_d2ui_hat] = fcn(c1, c2, c3, chi_t, ui_sig_1, ui_sig_2, ui_sig_3, ...
                                                                                        ui_sig_4, ui_sig_5, ui_sig_6, dui_hat, d2ui_hat)
d_d2ui_hat = -chi_t .* c1 * ui_sig_1(:) - (1 - chi_t) .* c1 * ui_sig_2(:);
d_dui_hat = -chi_t .* c2 * ui_sig_3(:) - (1 - chi_t) .* c2 * ui_sig_4(:) + d2ui_hat(:);
d_ui_hat = -chi_t .* c3 * ui_sig_5(:) - (1 - chi_t) .* c3 * ui_sig_6(:) + dui_hat(:);

== matlab function sim_tcst_2024_att_ctrl/cal sig12 ==
  data: x input; z output; y input
function z = fcn(x, y)
z = x(:) .* sign(y(:));

== matlab function sim_tcst_2024_att_ctrl/cal sig13 ==
  data: x input; z output; y input
function z = fcn(x, y)
z = x(:) .* sign(y(:));

== matlab function sim_tcst_2024_att_ctrl/cal sig14 ==
  data: x input; z output; y input
function z = fcn(x, y)
z = x(:) .* sign(y(:));

== matlab function sim_tcst_2024_att_ctrl/cal sig15 ==
  data: x input; z output; y input
function z = fcn(x, y)
z = x(:) .* sign(y(:));

== matlab function sim_tcst_2024_att_ctrl/cal sig16 ==
  data: x input; z output; y input
function z = fcn(x, y)
z = x(:) .* sign(y(:));

== matlab function sim_tcst_2024_att_ctrl/cal sig17 ==
  data: x input; z output; y input
function z = fcn(x, y)
z = x(:) .* sign(y(:));

== matlab function sim_tcst_2024_att_ctrl/choose ui agent 3 ==
  data: x input; y output
function y = fcn(x)
iiuav = 3;
y = x(:,iiuav);

== matlab function sim_tcst_2024_att_ctrl/trans to column17 ==
  data: x input; y output
function y = fcn(x)
y = x(:);

== matlab function sim_tcst_2024_att_ctrl/trans to column18 ==
  data: x input; y output
function y = fcn(x)
y = x(:);

== matlab function sim_tcst_2024_att_ctrl/trans to column19 ==
  data: x input; y output
function y = fcn(x)
y = x(:);

== matlab function sim_tcst_2024_att_ctrl/trans to column20 ==
  data: x input; y output
function y = fcn(x)
y = x(:);

== matlab function sim_tcst_2024_att_ctrl/trans to column21 ==
  data: x input; y output
function y = fcn(x)
y = x(:);

== matlab function sim_tcst_2024_att_ctrl/trans to column22 ==
  data: x input; y output
function y = fcn(x)
y = x(:);

== matlab function sim_tcst_2024_att_ctrl/cal d_theta_hat3 ==
  data: c1 input; d_ui_hat output; d_dui_hat output; d_d2ui_hat output; c2 input; c3 input; chi_t input; ui_sig_1 input; ui_sig_2 input; ui_sig_3 input; ui_sig_4 input; ui_sig_5 input; ui_sig_6 input; dui_hat input; d2ui_hat input
function [d_ui_hat, d_dui_hat, d_d2ui_hat] = fcn(c1, c2, c3, chi_t, ui_sig_1, ui_sig_2, ui_sig_3, ...
                                                                                        ui_sig_4, ui_sig_5, ui_sig_6, dui_hat, d2ui_hat)
d_d2ui_hat = -chi_t .* c1 * ui_sig_1(:) - (1 - chi_t) .* c1 * ui_sig_2(:);
d_dui_hat = -chi_t .* c2 * ui_sig_3(:) - (1 - chi_t) .* c2 * ui_sig_4(:) + d2ui_hat(:);
d_ui_hat = -chi_t .* c3 * ui_sig_5(:) - (1 - chi_t) .* c3 * ui_sig_6(:) + dui_hat(:);

== matlab function sim_tcst_2024_att_ctrl/cal sig18 ==
  data: x input; z output; y input
function z = fcn(x, y)
z = x(:) .* sign(y(:));

== matlab function sim_tcst_2024_att_ctrl/depart err_Ri_bar 2 ==
  data: y output; x input
function y = fcn(x)
y = x(:,2);

end

== matlab function sim_tcst_2024_att_ctrl/cal sig19 ==
  data: x input; z output; y input
function z = fcn(x, y)
z = x(:) .* sign(y(:));

== matlab function sim_tcst_2024_att_ctrl/cal sig20 ==
  data: x input; z output; y input
function z = fcn(x, y)
z = x(:) .* sign(y(:));

== matlab function sim_tcst_2024_att_ctrl/cal sig21 ==
  data: x input; z output; y input
function z = fcn(x, y)
z = x(:) .* sign(y(:));

== matlab function sim_tcst_2024_att_ctrl/cal sig22 ==
  data: x input; z output; y input
function z = fcn(x, y)
z = x(:) .* sign(y(:));

== matlab function sim_tcst_2024_att_ctrl/process velocity ==
  data: T0 input; T1 input; T2 input; PZ0 input; PZ1 input; R0 input; R1 input; Rx2 input; Ry2 input; Rz2 input; t input; V_init_out output
function V_init_out = fcn(T0, T1, T2, PZ0, PZ1, R0, R1, Rx2, Ry2, Rz2, t)
V_init_out = zeros(3, 1);
if t < T1 + 1e-05
    V_init_out(1, 1) = ( cos( ( 2 * pi * ( t - T0 ) ) / ( T0 - T1 ) ) * ( R0 - R1 ) ) / ( T0 - T1 ) ...
                                    - ( 2 * pi * sin( ( 2 * pi * ( t - T0 ) ) / ( T0 - T1 ) ) * ( R0 + ( ( R0 - R1 ) * ( t - T0 ) ) / ( T0 - T1 ) ) ) / ( T0 - T1 );
    V_init_out(2, 1) = ( sin( ( 2 * pi * ( t - T0 ) ) / ( T0 - T1 ) ) * ( R0 - R1 ) ) / ( T0 - T1 ) ...
                                    + ( 2 * pi * cos( ( 2 * pi * ( t - T0 ) ) / ( T0 - T1 ) ) * ( R0 + ( ( R0 - R1 ) * ( t - T0 ) ) / ( T0 - T1 ) ) ) / ( T0 - T1 );
    V_init_out(3, 1) = ( PZ0 - PZ1 ) / ( T0 - T1 );
else
    V_init_out(1, 1) = ( 2 * Rx2 * pi * sin( ( 2 * pi * ( t - T1 ) ) / ( T1 - T2 ) ) ) / ( T1 - T2 );
    V_init_out(2, 1) = ( 4 * Ry2 * pi * cos( ( 4 * pi * ( t - T1 ) ) / ( T1 - T2 ) ) ) / ( T1 - T2 );
    V_init_out(3, 1) = - ( 4 * Rz2 * pi * cos( ( 4 * pi * ( t - T1 ) ) / ( T1 - T2 ) ) ) / ( T1 - T2 );
end

== matlab function sim_tcst_2024_att_ctrl/cal sig23 ==
  data: x input; z output; y input
function z = fcn(x, y)
z = x(:) .* sign(y(:));

== matlab function sim_tcst_2024_att_ctrl/choose ui agent 4 ==
  data: x input; y output
function y = fcn(x)
iiuav = 4;
y = x(:,iiuav);

== matlab function sim_tcst_2024_att_ctrl/trans to column23 ==
  data: x input; y output
function y = fcn(x)
y = x(:);

== matlab function sim_tcst_2024_att_ctrl/trans to column24 ==
  data: x input; y output
function y = fcn(x)
y = x(:);

== matlab function sim_tcst_2024_att_ctrl/trans to column25 ==
  data: x input; y output
function y = fcn(x)
y = x(:);

== matlab function sim_tcst_2024_att_ctrl/trans to column26 ==
  data: x input; y output
function y = fcn(x)
y = x(:);

== matlab function sim_tcst_2024_att_ctrl/trans to column27 ==
  data: x input; y output
function y = fcn(x)
y = x(:);

== matlab function sim_tcst_2024_att_ctrl/trans to column28 ==
  data: x input; y output
function y = fcn(x)
y = x(:);

== matlab function sim_tcst_2024_att_ctrl/cal d_theta_hat4 ==
  data: c1 input; d_ui_hat output; d_dui_hat output; d_d2ui_hat output; c2 input; c3 input; chi_t input; ui_sig_1 input; ui_sig_2 input; ui_sig_3 input; ui_sig_4 input; ui_sig_5 input; ui_sig_6 input; dui_hat input; d2ui_hat input
function [d_ui_hat, d_dui_hat, d_d2ui_hat] = fcn(c1, c2, c3, chi_t, ui_sig_1, ui_sig_2, ui_sig_3, ...
                                                                                        ui_sig_4, ui_sig_5, ui_sig_6, dui_hat, d2ui_hat)
d_d2ui_hat = -chi_t .* c1 * ui_sig_1(:) - (1 - chi_t) .* c1 * ui_sig_2(:);
d_dui_hat = -chi_t .* c2 * ui_sig_3(:) - (1 - chi_t) .* c2 * ui_sig_4(:) + d2ui_hat(:);
d_ui_hat = -chi_t .* c3 * ui_sig_5(:) - (1 - chi_t) .* c3 * ui_sig_6(:) + dui_hat(:);

== matlab function sim_tcst_2024_att_ctrl/cal sig24 ==
  data: x input; z output; y input
function z = fcn(x, y)
z = x(:) .* sign(y(:));

== matlab function sim_tcst_2024_att_ctrl/cal sig25 ==
  data: x input; z output; y input
function z = fcn(x, y)
z = x(:) .* sign(y(:));

== matlab function sim_tcst_2024_att_ctrl/cal sig26 ==
  data: x input; z output; y input
function z = fcn(x, y)
z = x(:) .* sign(y(:));

== matlab function sim_tcst_2024_att_ctrl/cal sig27 ==
  data: x input; z output; y input
function z = fcn(x, y)
z = x(:) .* sign(y(:));

== matlab function sim_tcst_2024_att_ctrl/cal sig28 ==
  data: x input; z output; y input
function z = fcn(x, y)
z = x(:) .* sign(y(:));

== matlab function sim_tcst_2024_att_ctrl/cal sig29 ==
  data: x input; z output; y input
function z = fcn(x, y)
z = x(:) .* sign(y(:));

== matlab function sim_tcst_2024_att_ctrl/choose ui agent 5 ==
  data: x input; y output
function y = fcn(x)
iiuav = 5;
y = x(:,iiuav);

== matlab function sim_tcst_2024_att_ctrl/trans to column29 ==
  data: x input; y output
function y = fcn(x)
y = x(:);
